simulink library "sm_excv_track_lib"  (R2023a)
settings: Solver=VariableStepAuto  StartTime=0.0  StopTime=10.0  RelTol=1e-3
undefined symbols (not defined in the file): Excv, L1, L10, L11, L12, L13, L14, L15, L16, L17, L18, L19, L2, L20, L21, L22, L23, L24, L25, L26, L27, L28, L29, L3, L30, L31, L32, L33, L34, L35, L36, L37, L38, L39, L4, L40, L41, L42, L43, L44, L45, L46, L5, L6, L7, L8, L9, track_joint_targets
libraries: sm_tracked_vehicle_lib x92
(part 1 of 3)
settings Model: Creator=smiller  LastModifiedBy=smiller

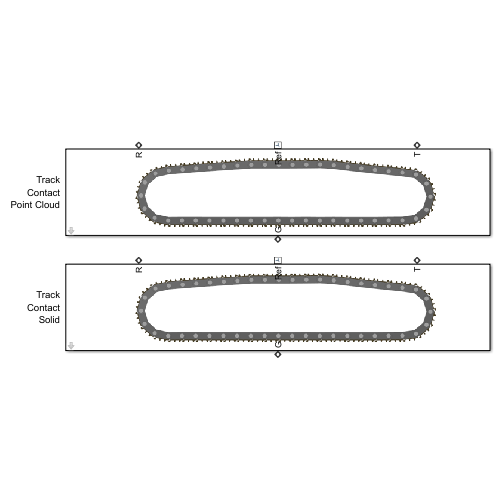
[thumbnail: Simulink's stored preview of the top-level diagram]
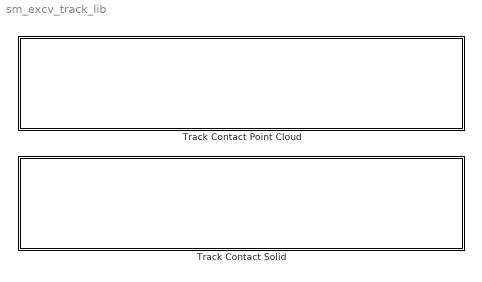
== system sm_excv_track_lib ==
  Track Contact Point Cloud : Subsystem  mask(Segmented Track with Point Cloud){chain_wid=Excv.Chain.chain_wid, chain_seg_m=Excv.Chain.link_m, chain_seg_cg=Excv.Chain.link_cg, chain_seg_moi=Excv.Chain.link_moi, chain_seg_poi=Excv.Chain.link_poi, plate_h=Excv.Chain.plate_h, plate_xc=Excv.Chain.plate_xc, plate_thk=Excv.Chain.plate_thk, pin_sep=Excv.Chain.pin_sep, plate_ang=Excv.Chain.plate_ang, plate_clr=Excv.Chain.plate_clr, plate_opc=Excv.Chain.plate_opc, pin_len=Excv.Chain.pin_len, pin_rad=Excv.Chain.pin_rad, pin_clr=Excv.Chain.pin_clr, pin_opc=Excv.Chain.pin_opc, shoe_xc=Excv.Shoe.xc, shoe_w=Excv.Shoe.w, shoe_m=Excv.Shoe.mass, shoe_cg=Excv.Shoe.cg, shoe_moi=Excv.Shoe.moi, shoe_poi=Excv.Shoe.poi, shoe_clr=Excv.Shoe.clr, shoe_opc=Excv.Shoe.opc, jointTargets=track_joint_targets, chainDamping=Excv.Chain.damping, ptcld_shoe=Excv.Shoe.ground_contact.ptcld.pts, ptcld_shoe_rad=Excv.Shoe.ground_contact.ptcld.rad, ptcld_shoe_clr=Excv.Shoe.ground_contact.ptcld.clr, ptcld_shoe_opc=Excv.Shoe.ground_contact.ptcld.opc, chain_to_roller_clr=Excv.Chain.roller_contact.clr, chain_to_roller_opc=Excv.Chain.roller_contact.opc, chain_to_teeth_clr=Excv.Chain.teeth_contact.clr, chain_to_teeth_opc=Excv.Chain.teeth_contact.opc}
      mask prompts: chain_wid "Width (m)"; chain_seg_m "Mass (kg)"; chain_seg_cg "CG [x y z] (kg)"; chain_seg_moi "Moments of Inertia [Ixx Iyy Izz] (kg*m^2)"; chain_seg_poi "Products of Inertia [Iyz Ixz Ixy] (kg*m^2)"; plate_h "Height (m)"; plate_xc "Extrusion [x y] (m)"; plate_thk "Thickness (m)"; pin_sep "Pin Separation (m)"; plate_ang "Angle (deg)"; plate_clr "Color [R G B] (0-1)"; plate_opc "Opacity (0-1)"; pin_len "Pin Length (m)"; pin_rad "Pin Radius (m)"; pin_clr "Pin Color [R G B] (0-1)"; pin_opc "Opacity (0-1)"; shoe_xc "Extrusion Profile [x y] (m)"; shoe_w "Width (m)"; shoe_m "Mass (kg)"; shoe_cg "CG [x y z ] (m)"; shoe_moi "Moments of Inertia [Ixx Iyy Izz] (kg*m^2)"; shoe_poi "Products of Inertia [Iyz Izx Ixy] (kg*m^2)"; shoe_clr "Color [R G B] (0-1)"; shoe_opc "Opacity (0-1)"; jointTargets "Joint Targets (structure)"; chainDamping "Joint Damping N*m/(deg/s)"; ptcld_shoe "Points [x y z] (m)"; ptcld_shoe_rad "Radius (m)"; ptcld_shoe_clr "Color [R G B] (0-1)"; ptcld_shoe_opc "Opacity (0-1)"; chain_to_roller_clr "Color [R G B] (0-1)"; chain_to_roller_opc "Opacity (0-1)"; chain_to_teeth_clr "Color [R G B] (0-1)"; chain_to_teeth_opc "Opacity (0-1)"
      mask help: Models a segmented track. Contact geometry in chain enables contact modeling with sprocket, rollers, and idler. Contact geometry (point cloud) in shoe enables contact with the ground.
      mask init:
      | for i = 1:size(jointTargets,1)
      |     blknum = pad(num2str(i),2,"left","0");
      |     blkname = [gcb '/Seg ' blknum];
      |     set_param(blkname,'posTgtSpecify',jointTargets{i,1});
      |     set_param(blkname,'posTgtPriority',jointTargets{i,2});
      |     set_param(blkname,'PositionTargetValue',num2str(jointTargets{i,3}));
      | end
      mask DialogControl cont_seg Prompt: Segment
      mask DialogControl cont_plates Prompt: Plates
      mask DialogControl cont_pin Prompt: Pin
      mask DialogControl cont_shoe Prompt: Shoe
      mask DialogControl cont_track_assembly Prompt: Assembly
      mask DialogControl cont_contact_geo Prompt: Contact Geometry
      mask DialogControl cont_shoe_plate Prompt: Shoe Plate Point Cloud
      mask DialogControl cont_chain_to_roller Prompt: Chain to Roller
      mask DialogControl cont_chain_to_teeth Prompt: Chain to Teeth
      mask Display: image('sm_excv_track_segments_sideview_IMAGE.png')
  Track Contact Solid : Subsystem  mask(Segmented Track with Brick Solid Contact Geometry){chain_wid=Excv.Chain.chain_wid, chain_seg_m=Excv.Chain.link_m, chain_seg_cg=Excv.Chain.link_cg, chain_seg_moi=Excv.Chain.link_moi, chain_seg_poi=Excv.Chain.link_poi, plate_h=Excv.Chain.plate_h, plate_xc=Excv.Chain.plate_xc, plate_thk=Excv.Chain.plate_thk, pin_sep=Excv.Chain.pin_sep, plate_ang=Excv.Chain.plate_ang, plate_clr=Excv.Chain.plate_clr, plate_opc=Excv.Chain.plate_opc, pin_len=Excv.Chain.pin_len, pin_rad=Excv.Chain.pin_rad, pin_clr=Excv.Chain.pin_clr, pin_opc=Excv.Chain.pin_opc, shoe_xc=Excv.Shoe.xc, shoe_w=Excv.Shoe.w, shoe_m=Excv.Shoe.mass, shoe_cg=Excv.Shoe.cg, shoe_moi=Excv.Shoe.moi, shoe_poi=Excv.Shoe.poi, shoe_clr=Excv.Shoe.clr, shoe_opc=Excv.Shoe.opc, jointTargets=track_joint_targets, chainDamping=Excv.Chain.damping, shoe_plate_h=Excv.Shoe.pad_h, shoe_plate_l=Excv.Shoe.l, shoe_plate_contact_clr=Excv.Shoe.ground_contact.plate_solid.clr, shoe_plate_contact_opc=Excv.Shoe.ground_contact.plate_solid.opc, chain_to_roller_clr=Excv.Chain.roller_contact.clr, chain_to_roller_opc=Excv.Chain.roller_contact.opc, chain_to_teeth_clr=Excv.Chain.teeth_contact.clr, chain_to_teeth_opc=Excv.Chain.teeth_contact.opc}
      mask prompts: chain_wid "Width (m)"; chain_seg_m "Mass (kg)"; chain_seg_cg "CG [x y z] (kg)"; chain_seg_moi "Moments of Inertia [Ixx Iyy Izz] (kg*m^2)"; chain_seg_poi "Products of Inertia [Iyz Ixz Ixy] (kg*m^2)"; plate_h "Height (m)"; plate_xc "Extrusion [x y] (m)"; plate_thk "Thickness (m)"; pin_sep "Pin Separation (m)"; plate_ang "Angle (deg)"; plate_clr "Color [R G B] (0-1)"; plate_opc "Opacity (0-1)"; pin_len "Pin Length (m)"; pin_rad "Pin Radius (m)"; pin_clr "Pin Color [R G B] (0-1)"; pin_opc "Opacity (0-1)"; shoe_xc "Extrusion Profile [x y] (m)"; shoe_w "Width (m)"; shoe_m "Mass (kg)"; shoe_cg "CG [x y z ] (m)"; shoe_moi "Moments of Inertia [Ixx Iyy Izz] (kg*m^2)"; shoe_poi "Products of Inertia [Iyz Izx Ixy] (kg*m^2)"; shoe_clr "Color [R G B] (0-1)"; shoe_opc "Opacity (0-1)"; jointTargets "Joint Targets (structure)"; chainDamping "Joint Damping N*m/(deg/s)"; shoe_plate_h "Pad Height (m)"; shoe_plate_l "Pad Length (m)"; shoe_plate_contact_clr "Color [R G B] (0-1)"; shoe_plate_contact_opc "Opacity (0-1)"; chain_to_roller_clr "Color [R G B] (0-1)"; chain_to_roller_opc "Opacity (0-1)"; chain_to_teeth_clr "Color [R G B] (0-1)"; chain_to_teeth_opc "Opacity (0-1)"
      mask help: Models a segmented track. Contact geometry in chain enables contact modeling with sprocket, rollers, and idler. Contact geometry (brick solid) in shoe enables contact with the ground.
      mask init: same as sm_excv_track_lib/Track Contact Point Cloud
      mask DialogControl cont_seg Prompt: Segment
      mask DialogControl cont_plates Prompt: Plates
      mask DialogControl cont_pin Prompt: Pin
      mask DialogControl cont_shoe Prompt: Shoe
      mask DialogControl cont_track_assembly Prompt: Assembly
      mask DialogControl cont_contact Prompt: Contact Geometry
      mask DialogControl cont_shoe_plate_solid Prompt: Shoe Plate Solid
      mask DialogControl cont_chain_to_roller Prompt: Chain to Roller
      mask DialogControl cont_chain_to_teeth Prompt: Chain to Teeth
      mask Display: image('sm_excv_track_segments_sideview_IMAGE.png')
